simulink model "binNeural"  (R2012b)
settings: Solver=FixedStepDiscrete  StartTime=0.0  StopTime=10.0  FixedStep=0.001  RelTol=1e-3
settings Model: BufferReuse=off  Creator=gilja  LastModifiedBy=Chethan
settings SolverCC: EnableConcurrentExecution=on  ConcurrentTasks=on
settings DataIOCC: SaveOutput=off  SignalLogging=off  DSMLogging=off  SaveTime=off
settings OptimizationCC: InlineParams=on  InlineInvariantSignals=on  OptimizeBlockIOStorage=off  BufferReuse=off  ExpressionFolding=off  LocalBlockOutputs=off
settings HardwareCC: ProdIntDivRoundTo=Zero  ProdEndianess=LittleEndian  ProdHWDeviceType=Generic->32-bit x86 compatible
settings ModelReferenceCC: ModelReferenceMinAlgLoopOccurrences=on
settings RTWCC: SystemTargetFile=xpctarget.tlc  TemplateMakefile=xpc_default_tmf  Description=xPC Target  ProcessScript=xpctarget_make_rtw_hook  RTWCompilerOptimization=On
settings CodeAppCC: MaxIdLength=62
settings xpcTargetCC: TargetFcnLib=ansi_tfl_table_tmw.mat  CodeReplacementLibrary=XPC_BLAS  ParMdlRefBuildCompliant=on  ConcurrentExecutionCompliant=on  CombineSignalStateStructs=off  GRTInterface=on  xPCTaskExecutionProfile=on  xPCRL32EventNumber=5000  xPCisDownloadable=off  xPCLoadParamSetFile=off  xPCConcurrentTasks=off  xPCEnableSFAnimation=off

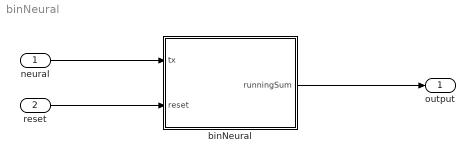
== system binNeural ==
  neural : Inport
  reset : Inport  Port=2
  binNeural : MATLAB Function  TreatAsAtomicUnit=on
  output : Outport  BusOutputAsStruct=on
  wires:
  binNeural/1(runningSum) -> output/1
  neural/1 -> binNeural/1(tx)
  reset/1 -> binNeural/2(reset)

== matlab function binNeural/binNeural ==
  data: tx input double size=[1 2*DecoderConstants.NUM_CHANNELS_PER_ARRAY]; reset input double; runningSum output size=[1 2*DecoderConstants.NUM_CHANNELS_PER_ARRAY]
function runningSum = binNeural(tx, reset)
    persistent binnedOut
    if isempty(binnedOut)
        binnedOut = double(tx);
    end
    
    if reset
        binnedOut = double(tx);
    else
        binnedOut = binnedOut + double(tx);
    end
    
    runningSum = binnedOut;
